simulink model "dspstfft_audio"  (Simulink 7.2)
settings: Solver=FixedStepDiscrete  StartTime=0.0  StopTime=inf  RelTol=1e-3
undefined symbols (not defined in the file or in its folder): jet
libraries: dspbuff3 x2, dspsnks4 x2, dspsrcs4 x1, dspmisc x1, dspspect3 x1, dspmtrx3 x1, dspmathops x1
settings Model: Creator=The MathWorks Inc.  ExtModeAutoUpdateStatusClock=off
settings DataIOCC: SaveOutput=off  SaveTime=off  SignalLoggingName=logsOut
settings OptimizationCC: BlockReduction=off  BooleanDataType=off  InlineInvariantSignals=on  InitFltsAndDblsToZero=on
settings DebuggingCC: SignalResolutionControl=TryResolveAllWithWarning  SolverPrmCheckMsg=none  MultiTaskDSMMsg=warning  MultiTaskCondExecSysMsg=none  StrictBusMsg=None
settings HardwareCC: ProdHWDeviceType=Specified
settings RTWCC: IncludeERTFirstTime=on

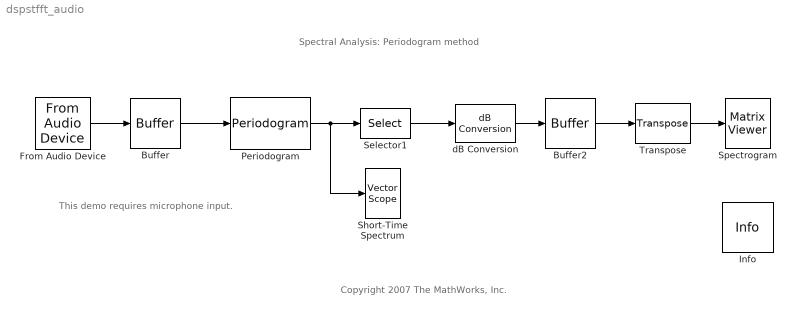
== system dspstfft_audio ==
  note: This demo requires microphone input.
  note: Spectral Analysis: Periodogram method
  note: Copyright 2007 The MathWorks, Inc.
  Buffer : dspbuff3/Buffer  N=128  V=48  ic=0
  Buffer2 : dspbuff3/Buffer  N=48  V=46  ic=-70
  From Audio Device : dspsrcs4/From Audio Device  DialogController=dspDDGCreate  DialogControllerArgs=DataTag0  deviceName=Default  numChannels=1  sampleRate=8000  deviceDatatype=16-bit integer  autoBufferSize=on  bufferSize=4096  queueDuration=1.0  frameSize=256  outputDatatype=double
  Info : dspmisc/Info  SystemSampleTime=-1
  Periodogram : dspspect3/Periodogram  SystemSampleTime=-1  wintype=Hamming  Rs=50  beta=5  winsamp=Periodic  inheritFFT=on  fftsize=128  navg=2
  Selector1 : Selector  InputPortWidth=128  IndexOptions=Index vector (dialog)  Indices=1:64  OutputSizes=1
  Short-Time Spectrum : dspsnks4/Vector Scope  DialogController=dspdialog.VectorScope  DialogControllerArgs=DataTag1  ScopeProperties=on  Domain=Frequency  HorizSpan=1  DisplayProperties=off  AxisGrid=off  Memory=off  FrameNumber=off  AxisLegend=off  AxisZoom=off  OpenScopeAtSimStart=on  OpenScopeImmediately=off  FigPos=[80 110 380 320]  AxisProperties=off  XUnits=Hertz  XRange=[0...Fs/2]  InheritXIncr=off  XIncr=1/8000  XLabel=Samples  XLimit=Auto  XMin=0  XMax=1  XStart=0  YUnits=dB  YLabel=Magnitude, dB  LineProperties=off
      settings: YMin=-59.7576717829863  YMax=9.71199466608513
  Spectrogram : dspsnks4/Matrix Viewer  DialogController=dspdialog.MatrixViewer  DialogControllerArgs=DataTag2  ImageParams=off  CMapStr=jet(256)  AxisColorbar=on  AxisParams=off  AxisOrigin=Lower left corner  XLabel=Time Index  YLabel=Frequency Index  ZLabel=dB Magnitude  FigPos=[468 110 380 320]  AxisZoom=off
      settings: YMin=-70  YMax=15
  Transpose : dspmtrx3/Transpose  SystemSampleTime=-1  Hermitian=off  overflowFlag=on
  dB Conversion : dspmathops/dB Conversion  SystemSampleTime=-1  dBtype=dB  intype=Amplitude  R=1  fuzz=on
  wires:
  Buffer/1 -> Periodogram/1
  From Audio Device/1 -> Buffer/1
  Selector1/1 -> dB Conversion/1
  dB Conversion/1 -> Buffer2/1
  Buffer2/1 -> Transpose/1
  Transpose/1 -> Spectrogram/1
  Periodogram/1 -> Selector1/1, Short-Time Spectrum/1
